simulink model "rvs_testing"  (R2016a)
settings: Solver=ode45  StartTime=0.0  StopTime=10.0  RelTol=1e-3
libraries: rvs x4
settings Model: Creator=Arthur  LastModifiedBy=aeagr
settings DataIOCC: LimitDataPoints=on  SaveFormat=Array
settings DebuggingCC: SolverPrmCheckMsg=warning
settings HardwareCC: ProdBitPerPointer=32  ProdLargestAtomicFloat=None  ProdIntDivRoundTo=Undefined  ProdEndianess=Unspecified  ProdWordSize=32  ProdHWDeviceType=32-bit Generic
settings ModelReferenceCC: PropagateSignalLabelsOutOfModel=off
settings ConfigComp: CovModelRefEnable=Off  CovSFcnEnable=off

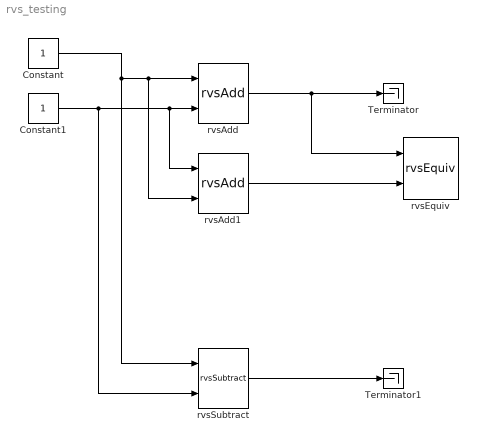
== system rvs_testing ==
  Constant : Constant
  Constant1 : Constant
  Terminator : Terminator
  Terminator1 : Terminator
  rvsAdd : rvs/rvsAdd
  rvsAdd1 : rvs/rvsAdd
  rvsEquiv : rvs/rvsEquiv
  rvsSubtract : rvs/rvsSubtract
  wires:
  Constant1/1 -> rvsSubtract/2, rvsAdd1/1, rvsAdd/2
  rvsAdd/1 -> rvsEquiv/1, Terminator/1
  Constant/1 -> rvsSubtract/1, rvsAdd1/2, rvsAdd/1
  rvsSubtract/1 -> Terminator1/1
  rvsAdd1/1 -> rvsEquiv/2
